simulink model "gm_max_frequency_index"  (R2020a)
settings: Solver=FixedStepDiscrete  StartTime=0.0  StopTime=1e-2  RelTol=1e-3
model workspace (MAT data in the model file):
  amplitud = 2047
  fft_length = 32
  samples_per_period = 3
  sampling_time = 1e-06
libraries: simulink x384, dspsrcs4 x1, dsphdlxfrm x1, dspstat3 x1, hdlsllib x1
(part 2 of 18)

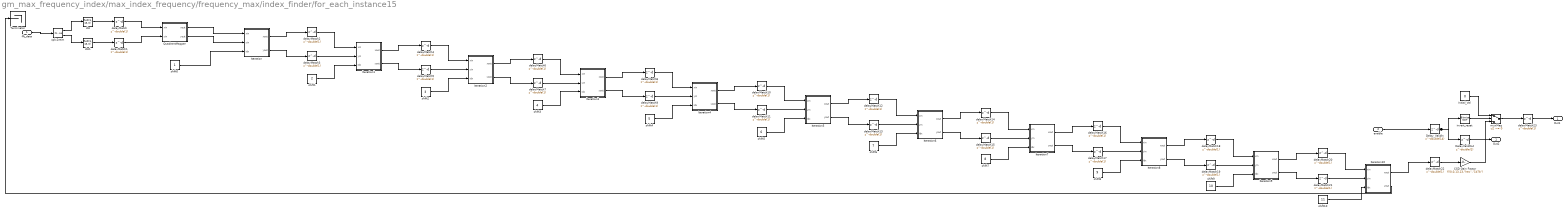
== system gm_max_frequency_index/max_index_frequency/frequency_max/index_finder/for_each_instance15 ==
  fft_data : Inport  OutDataTypeStr=fixdt(1, 12, 0)  PortDimensions=1  SampleTime=3.2e-05
      settings: SignalType=complex
  enable : Inport  Port=2  OutDataTypeStr=boolean  PortDimensions=1  SampleTime=3.2e-05
  CSD Gain Factor : Gain  Gain="fi(0,0,13,13,\"hex\",\"1b7b\")"  ParamDataTypeStr=fixdt(0, 13, 13)  OutDataTypeStr=fixdt(1, 13, 0)  SampleTime=3.2e-05
  DelayValidOut : Delay  DelayLength=double(1)  InitialCondition=0  SampleTime=3.2e-05
  Delay_ValidIn : Delay  DelayLength=double(14)  InitialCondition=0  SampleTime=3.2e-05
  Initial_Val : Constant  Value=0  OutDataTypeStr=fixdt(1, 13, 0)  SampleTime=3.2e-05
  Iteration : Subsystem
  Iteration1 : Subsystem
  Iteration10 : Subsystem
  Iteration2 : Subsystem
  Iteration3 : Subsystem
  Iteration4 : Subsystem
  Iteration5 : Subsystem
  Iteration6 : Subsystem
  Iteration7 : Subsystem
  Iteration8 : Subsystem
  Iteration9 : Subsystem
  QuadrantMapper : Subsystem
  Terminator : Terminator
  cplx2reim : ComplexToRealImag  SampleTime=3.2e-05
  delayMatch{,1..23} (24 alike) : Delay  DelayLength=double(1)  InitialCondition=0  SampleTime=3.2e-05
  dtc : DataTypeConversion  OutDataTypeStr=fixdt(1, 13, 0)  SampleTime=3.2e-05
  dtc1 : DataTypeConversion  OutDataTypeStr=fixdt(1, 13, 0)  SampleTime=3.2e-05
  invert_reset : simulink/Logic and Bit Operations/Bitwise Operator  logicop=NOT  UseBitMask=off  BitMask=double(0)  BitMaskRealWorld=Real World Value
  muxMag : Switch  Criteria=u2 ~= 0  Threshold=double(0)  OutDataTypeStr=fixdt(1, 13, 0)  SampleTime=3.2e-05
  shift0 : Constant  VectorParams1D=off  OutDataTypeStr=fixdt(0, 5, 0)  SampleTime=3.2e-05
  shift1 : Constant  Value=2  VectorParams1D=off  OutDataTypeStr=fixdt(0, 5, 0)  SampleTime=3.2e-05
  shift10 : Constant  Value=11  VectorParams1D=off  OutDataTypeStr=fixdt(0, 5, 0)  SampleTime=3.2e-05
  shift2 : Constant  Value=3  VectorParams1D=off  OutDataTypeStr=fixdt(0, 5, 0)  SampleTime=3.2e-05
  shift3 : Constant  Value=4  VectorParams1D=off  OutDataTypeStr=fixdt(0, 5, 0)  SampleTime=3.2e-05
  shift4 : Constant  Value=5  VectorParams1D=off  OutDataTypeStr=fixdt(0, 5, 0)  SampleTime=3.2e-05
  shift5 : Constant  Value=6  VectorParams1D=off  OutDataTypeStr=fixdt(0, 5, 0)  SampleTime=3.2e-05
  shift6 : Constant  Value=7  VectorParams1D=off  OutDataTypeStr=fixdt(0, 5, 0)  SampleTime=3.2e-05
  shift7 : Constant  Value=8  VectorParams1D=off  OutDataTypeStr=fixdt(0, 5, 0)  SampleTime=3.2e-05
  shift8 : Constant  Value=9  VectorParams1D=off  OutDataTypeStr=fixdt(0, 5, 0)  SampleTime=3.2e-05
  shift9 : Constant  Value=10  VectorParams1D=off  OutDataTypeStr=fixdt(0, 5, 0)  SampleTime=3.2e-05
  Out1 : Outport
  Out2 : Outport  Port=2  VectorParamsAs1DForOutWhenUnconnected=off
  wires:
  muxMag/1 -> delayMatch23/1
  invert_reset/1 -> muxMag/2
  CSD Gain Factor/1 -> muxMag/3
  Initial_Val/1 -> muxMag/1
  Iteration10/1(xout) -> delayMatch22/1
  shift10/1 -> Iteration10/3(idx)
  Iteration10/2(yout) -> Terminator/1
  Iteration9/2(yout) -> delayMatch21/1
  Iteration9/1(xout) -> delayMatch20/1
  shift9/1 -> Iteration9/3(idx)
  Iteration8/2(yout) -> delayMatch19/1
  Iteration8/1(xout) -> delayMatch18/1
  shift8/1 -> Iteration8/3(idx)
  Iteration7/2(yout) -> delayMatch17/1
  Iteration7/1(xout) -> delayMatch16/1
  shift7/1 -> Iteration7/3(idx)
  Iteration6/2(yout) -> delayMatch15/1
  Iteration6/1(xout) -> delayMatch14/1
  shift6/1 -> Iteration6/3(idx)
  Iteration5/2(yout) -> delayMatch13/1
  Iteration5/1(xout) -> delayMatch12/1
  shift5/1 -> Iteration5/3(idx)
  Iteration4/2(yout) -> delayMatch11/1
  Iteration4/1(xout) -> delayMatch10/1
  shift4/1 -> Iteration4/3(idx)
  Iteration3/2(yout) -> delayMatch9/1
  Iteration3/1(xout) -> delayMatch8/1
  shift3/1 -> Iteration3/3(idx)
  Iteration2/2(yout) -> delayMatch7/1
  Iteration2/1(xout) -> delayMatch6/1
  shift2/1 -> Iteration2/3(idx)
  Iteration1/2(yout) -> delayMatch5/1
  Iteration1/1(xout) -> delayMatch4/1
  shift1/1 -> Iteration1/3(idx)
  Iteration/2(yout) -> delayMatch3/1
  Iteration/1(xout) -> delayMatch2/1
  shift0/1 -> Iteration/3(idx)
  dtc1/1 -> delayMatch1/1
  dtc/1 -> delayMatch/1
  cplx2reim/2 -> dtc1/1
  cplx2reim/1 -> dtc/1
  enable/1 -> Delay_ValidIn/1
  fft_data/1 -> cplx2reim/1
  delayMatch23/1 -> Out1/1
  Delay_ValidIn/1 -> invert_reset/1, DelayValidOut/1
  QuadrantMapper/2(yout) -> Iteration/2(yin)
  QuadrantMapper/1(xout) -> Iteration/1(xin)
  delayMatch1/1 -> QuadrantMapper/2(yin)
  delayMatch/1 -> QuadrantMapper/1(xin)
  delayMatch22/1 -> CSD Gain Factor/1
  delayMatch21/1 -> Iteration10/2(yin)
  delayMatch20/1 -> Iteration10/1(xin)
  delayMatch19/1 -> Iteration9/2(yin)
  delayMatch18/1 -> Iteration9/1(xin)
  delayMatch17/1 -> Iteration8/2(yin)
  delayMatch16/1 -> Iteration8/1(xin)
  delayMatch15/1 -> Iteration7/2(yin)
  delayMatch14/1 -> Iteration7/1(xin)
  delayMatch13/1 -> Iteration6/2(yin)
  delayMatch12/1 -> Iteration6/1(xin)
  delayMatch11/1 -> Iteration5/2(yin)
  delayMatch10/1 -> Iteration5/1(xin)
  delayMatch9/1 -> Iteration4/2(yin)
  delayMatch8/1 -> Iteration4/1(xin)
  delayMatch7/1 -> Iteration3/2(yin)
  delayMatch6/1 -> Iteration3/1(xin)
  delayMatch5/1 -> Iteration2/2(yin)
  delayMatch4/1 -> Iteration2/1(xin)
  delayMatch3/1 -> Iteration1/2(yin)
  delayMatch2/1 -> Iteration1/1(xin)
  DelayValidOut/1 -> Out2/1

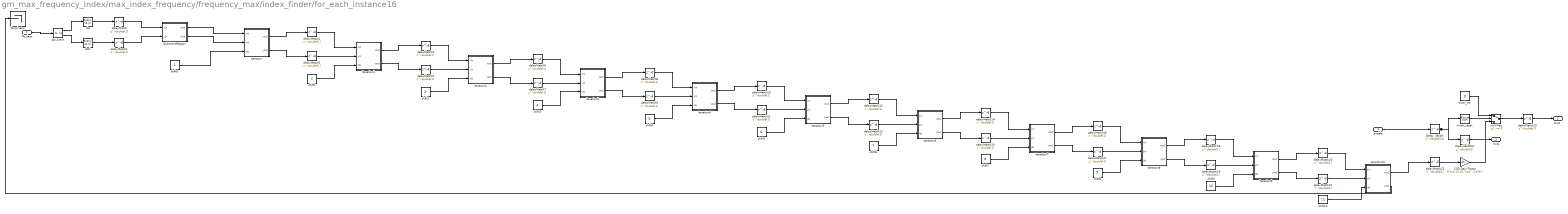
== system gm_max_frequency_index/max_index_frequency/frequency_max/index_finder/for_each_instance16 ==
  fft_data : Inport  OutDataTypeStr=fixdt(1, 12, 0)  PortDimensions=1  SampleTime=3.2e-05
      settings: SignalType=complex
  enable : Inport  Port=2  OutDataTypeStr=boolean  PortDimensions=1  SampleTime=3.2e-05
  CSD Gain Factor : Gain  Gain="fi(0,0,13,13,\"hex\",\"1b7b\")"  ParamDataTypeStr=fixdt(0, 13, 13)  OutDataTypeStr=fixdt(1, 13, 0)  SampleTime=3.2e-05
  DelayValidOut : Delay  DelayLength=double(1)  InitialCondition=0  SampleTime=3.2e-05
  Delay_ValidIn : Delay  DelayLength=double(14)  InitialCondition=0  SampleTime=3.2e-05
  Initial_Val : Constant  Value=0  OutDataTypeStr=fixdt(1, 13, 0)  SampleTime=3.2e-05
  Iteration : Subsystem
  Iteration1 : Subsystem
  Iteration10 : Subsystem
  Iteration2 : Subsystem
  Iteration3 : Subsystem
  Iteration4 : Subsystem
  Iteration5 : Subsystem
  Iteration6 : Subsystem
  Iteration7 : Subsystem
  Iteration8 : Subsystem
  Iteration9 : Subsystem
  QuadrantMapper : Subsystem
  Terminator : Terminator
  cplx2reim : ComplexToRealImag  SampleTime=3.2e-05
  delayMatch{,1..23} (24 alike) : Delay  DelayLength=double(1)  InitialCondition=0  SampleTime=3.2e-05
  dtc : DataTypeConversion  OutDataTypeStr=fixdt(1, 13, 0)  SampleTime=3.2e-05
  dtc1 : DataTypeConversion  OutDataTypeStr=fixdt(1, 13, 0)  SampleTime=3.2e-05
  invert_reset : simulink/Logic and Bit Operations/Bitwise Operator  logicop=NOT  UseBitMask=off  BitMask=double(0)  BitMaskRealWorld=Real World Value
  muxMag : Switch  Criteria=u2 ~= 0  Threshold=double(0)  OutDataTypeStr=fixdt(1, 13, 0)  SampleTime=3.2e-05
  shift0 : Constant  VectorParams1D=off  OutDataTypeStr=fixdt(0, 5, 0)  SampleTime=3.2e-05
  shift1 : Constant  Value=2  VectorParams1D=off  OutDataTypeStr=fixdt(0, 5, 0)  SampleTime=3.2e-05
  shift10 : Constant  Value=11  VectorParams1D=off  OutDataTypeStr=fixdt(0, 5, 0)  SampleTime=3.2e-05
  shift2 : Constant  Value=3  VectorParams1D=off  OutDataTypeStr=fixdt(0, 5, 0)  SampleTime=3.2e-05
  shift3 : Constant  Value=4  VectorParams1D=off  OutDataTypeStr=fixdt(0, 5, 0)  SampleTime=3.2e-05
  shift4 : Constant  Value=5  VectorParams1D=off  OutDataTypeStr=fixdt(0, 5, 0)  SampleTime=3.2e-05
  shift5 : Constant  Value=6  VectorParams1D=off  OutDataTypeStr=fixdt(0, 5, 0)  SampleTime=3.2e-05
  shift6 : Constant  Value=7  VectorParams1D=off  OutDataTypeStr=fixdt(0, 5, 0)  SampleTime=3.2e-05
  shift7 : Constant  Value=8  VectorParams1D=off  OutDataTypeStr=fixdt(0, 5, 0)  SampleTime=3.2e-05
  shift8 : Constant  Value=9  VectorParams1D=off  OutDataTypeStr=fixdt(0, 5, 0)  SampleTime=3.2e-05
  shift9 : Constant  Value=10  VectorParams1D=off  OutDataTypeStr=fixdt(0, 5, 0)  SampleTime=3.2e-05
  Out1 : Outport
  Out2 : Outport  Port=2  VectorParamsAs1DForOutWhenUnconnected=off
  wires:
  muxMag/1 -> delayMatch23/1
  invert_reset/1 -> muxMag/2
  CSD Gain Factor/1 -> muxMag/3
  Initial_Val/1 -> muxMag/1
  Iteration10/1(xout) -> delayMatch22/1
  shift10/1 -> Iteration10/3(idx)
  Iteration10/2(yout) -> Terminator/1
  Iteration9/2(yout) -> delayMatch21/1
  Iteration9/1(xout) -> delayMatch20/1
  shift9/1 -> Iteration9/3(idx)
  Iteration8/2(yout) -> delayMatch19/1
  Iteration8/1(xout) -> delayMatch18/1
  shift8/1 -> Iteration8/3(idx)
  Iteration7/2(yout) -> delayMatch17/1
  Iteration7/1(xout) -> delayMatch16/1
  shift7/1 -> Iteration7/3(idx)
  Iteration6/2(yout) -> delayMatch15/1
  Iteration6/1(xout) -> delayMatch14/1
  shift6/1 -> Iteration6/3(idx)
  Iteration5/2(yout) -> delayMatch13/1
  Iteration5/1(xout) -> delayMatch12/1
  shift5/1 -> Iteration5/3(idx)
  Iteration4/2(yout) -> delayMatch11/1
  Iteration4/1(xout) -> delayMatch10/1
  shift4/1 -> Iteration4/3(idx)
  Iteration3/2(yout) -> delayMatch9/1
  Iteration3/1(xout) -> delayMatch8/1
  shift3/1 -> Iteration3/3(idx)
  Iteration2/2(yout) -> delayMatch7/1
  Iteration2/1(xout) -> delayMatch6/1
  shift2/1 -> Iteration2/3(idx)
  Iteration1/2(yout) -> delayMatch5/1
  Iteration1/1(xout) -> delayMatch4/1
  shift1/1 -> Iteration1/3(idx)
  Iteration/2(yout) -> delayMatch3/1
  Iteration/1(xout) -> delayMatch2/1
  shift0/1 -> Iteration/3(idx)
  dtc1/1 -> delayMatch1/1
  dtc/1 -> delayMatch/1
  cplx2reim/2 -> dtc1/1
  cplx2reim/1 -> dtc/1
  enable/1 -> Delay_ValidIn/1
  fft_data/1 -> cplx2reim/1
  delayMatch23/1 -> Out1/1
  Delay_ValidIn/1 -> invert_reset/1, DelayValidOut/1
  QuadrantMapper/2(yout) -> Iteration/2(yin)
  QuadrantMapper/1(xout) -> Iteration/1(xin)
  delayMatch1/1 -> QuadrantMapper/2(yin)
  delayMatch/1 -> QuadrantMapper/1(xin)
  delayMatch22/1 -> CSD Gain Factor/1
  delayMatch21/1 -> Iteration10/2(yin)
  delayMatch20/1 -> Iteration10/1(xin)
  delayMatch19/1 -> Iteration9/2(yin)
  delayMatch18/1 -> Iteration9/1(xin)
  delayMatch17/1 -> Iteration8/2(yin)
  delayMatch16/1 -> Iteration8/1(xin)
  delayMatch15/1 -> Iteration7/2(yin)
  delayMatch14/1 -> Iteration7/1(xin)
  delayMatch13/1 -> Iteration6/2(yin)
  delayMatch12/1 -> Iteration6/1(xin)
  delayMatch11/1 -> Iteration5/2(yin)
  delayMatch10/1 -> Iteration5/1(xin)
  delayMatch9/1 -> Iteration4/2(yin)
  delayMatch8/1 -> Iteration4/1(xin)
  delayMatch7/1 -> Iteration3/2(yin)
  delayMatch6/1 -> Iteration3/1(xin)
  delayMatch5/1 -> Iteration2/2(yin)
  delayMatch4/1 -> Iteration2/1(xin)
  delayMatch3/1 -> Iteration1/2(yin)
  delayMatch2/1 -> Iteration1/1(xin)
  DelayValidOut/1 -> Out2/1

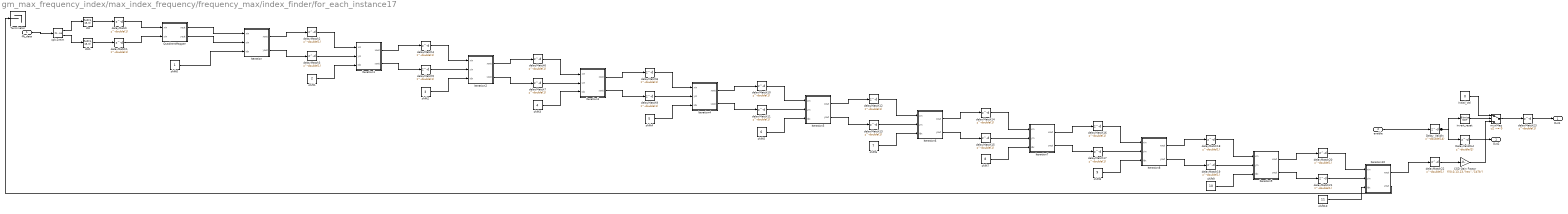
== system gm_max_frequency_index/max_index_frequency/frequency_max/index_finder/for_each_instance17 ==
  fft_data : Inport  OutDataTypeStr=fixdt(1, 12, 0)  PortDimensions=1  SampleTime=3.2e-05
      settings: SignalType=complex
  enable : Inport  Port=2  OutDataTypeStr=boolean  PortDimensions=1  SampleTime=3.2e-05
  CSD Gain Factor : Gain  Gain="fi(0,0,13,13,\"hex\",\"1b7b\")"  ParamDataTypeStr=fixdt(0, 13, 13)  OutDataTypeStr=fixdt(1, 13, 0)  SampleTime=3.2e-05
  DelayValidOut : Delay  DelayLength=double(1)  InitialCondition=0  SampleTime=3.2e-05
  Delay_ValidIn : Delay  DelayLength=double(14)  InitialCondition=0  SampleTime=3.2e-05
  Initial_Val : Constant  Value=0  OutDataTypeStr=fixdt(1, 13, 0)  SampleTime=3.2e-05
  Iteration : Subsystem
  Iteration1 : Subsystem
  Iteration10 : Subsystem
  Iteration2 : Subsystem
  Iteration3 : Subsystem
  Iteration4 : Subsystem
  Iteration5 : Subsystem
  Iteration6 : Subsystem
  Iteration7 : Subsystem
  Iteration8 : Subsystem
  Iteration9 : Subsystem
  QuadrantMapper : Subsystem
  Terminator : Terminator
  cplx2reim : ComplexToRealImag  SampleTime=3.2e-05
  delayMatch{,1..23} (24 alike) : Delay  DelayLength=double(1)  InitialCondition=0  SampleTime=3.2e-05
  dtc : DataTypeConversion  OutDataTypeStr=fixdt(1, 13, 0)  SampleTime=3.2e-05
  dtc1 : DataTypeConversion  OutDataTypeStr=fixdt(1, 13, 0)  SampleTime=3.2e-05
  invert_reset : simulink/Logic and Bit Operations/Bitwise Operator  logicop=NOT  UseBitMask=off  BitMask=double(0)  BitMaskRealWorld=Real World Value
  muxMag : Switch  Criteria=u2 ~= 0  Threshold=double(0)  OutDataTypeStr=fixdt(1, 13, 0)  SampleTime=3.2e-05
  shift0 : Constant  VectorParams1D=off  OutDataTypeStr=fixdt(0, 5, 0)  SampleTime=3.2e-05
  shift1 : Constant  Value=2  VectorParams1D=off  OutDataTypeStr=fixdt(0, 5, 0)  SampleTime=3.2e-05
  shift10 : Constant  Value=11  VectorParams1D=off  OutDataTypeStr=fixdt(0, 5, 0)  SampleTime=3.2e-05
  shift2 : Constant  Value=3  VectorParams1D=off  OutDataTypeStr=fixdt(0, 5, 0)  SampleTime=3.2e-05
  shift3 : Constant  Value=4  VectorParams1D=off  OutDataTypeStr=fixdt(0, 5, 0)  SampleTime=3.2e-05
  shift4 : Constant  Value=5  VectorParams1D=off  OutDataTypeStr=fixdt(0, 5, 0)  SampleTime=3.2e-05
  shift5 : Constant  Value=6  VectorParams1D=off  OutDataTypeStr=fixdt(0, 5, 0)  SampleTime=3.2e-05
  shift6 : Constant  Value=7  VectorParams1D=off  OutDataTypeStr=fixdt(0, 5, 0)  SampleTime=3.2e-05
  shift7 : Constant  Value=8  VectorParams1D=off  OutDataTypeStr=fixdt(0, 5, 0)  SampleTime=3.2e-05
  shift8 : Constant  Value=9  VectorParams1D=off  OutDataTypeStr=fixdt(0, 5, 0)  SampleTime=3.2e-05
  shift9 : Constant  Value=10  VectorParams1D=off  OutDataTypeStr=fixdt(0, 5, 0)  SampleTime=3.2e-05
  Out1 : Outport
  Out2 : Outport  Port=2  VectorParamsAs1DForOutWhenUnconnected=off
  wires:
  muxMag/1 -> delayMatch23/1
  invert_reset/1 -> muxMag/2
  CSD Gain Factor/1 -> muxMag/3
  Initial_Val/1 -> muxMag/1
  Iteration10/1(xout) -> delayMatch22/1
  shift10/1 -> Iteration10/3(idx)
  Iteration10/2(yout) -> Terminator/1
  Iteration9/2(yout) -> delayMatch21/1
  Iteration9/1(xout) -> delayMatch20/1
  shift9/1 -> Iteration9/3(idx)
  Iteration8/2(yout) -> delayMatch19/1
  Iteration8/1(xout) -> delayMatch18/1
  shift8/1 -> Iteration8/3(idx)
  Iteration7/2(yout) -> delayMatch17/1
  Iteration7/1(xout) -> delayMatch16/1
  shift7/1 -> Iteration7/3(idx)
  Iteration6/2(yout) -> delayMatch15/1
  Iteration6/1(xout) -> delayMatch14/1
  shift6/1 -> Iteration6/3(idx)
  Iteration5/2(yout) -> delayMatch13/1
  Iteration5/1(xout) -> delayMatch12/1
  shift5/1 -> Iteration5/3(idx)
  Iteration4/2(yout) -> delayMatch11/1
  Iteration4/1(xout) -> delayMatch10/1
  shift4/1 -> Iteration4/3(idx)
  Iteration3/2(yout) -> delayMatch9/1
  Iteration3/1(xout) -> delayMatch8/1
  shift3/1 -> Iteration3/3(idx)
  Iteration2/2(yout) -> delayMatch7/1
  Iteration2/1(xout) -> delayMatch6/1
  shift2/1 -> Iteration2/3(idx)
  Iteration1/2(yout) -> delayMatch5/1
  Iteration1/1(xout) -> delayMatch4/1
  shift1/1 -> Iteration1/3(idx)
  Iteration/2(yout) -> delayMatch3/1
  Iteration/1(xout) -> delayMatch2/1
  shift0/1 -> Iteration/3(idx)
  dtc1/1 -> delayMatch1/1
  dtc/1 -> delayMatch/1
  cplx2reim/2 -> dtc1/1
  cplx2reim/1 -> dtc/1
  enable/1 -> Delay_ValidIn/1
  fft_data/1 -> cplx2reim/1
  delayMatch23/1 -> Out1/1
  Delay_ValidIn/1 -> invert_reset/1, DelayValidOut/1
  QuadrantMapper/2(yout) -> Iteration/2(yin)
  QuadrantMapper/1(xout) -> Iteration/1(xin)
  delayMatch1/1 -> QuadrantMapper/2(yin)
  delayMatch/1 -> QuadrantMapper/1(xin)
  delayMatch22/1 -> CSD Gain Factor/1
  delayMatch21/1 -> Iteration10/2(yin)
  delayMatch20/1 -> Iteration10/1(xin)
  delayMatch19/1 -> Iteration9/2(yin)
  delayMatch18/1 -> Iteration9/1(xin)
  delayMatch17/1 -> Iteration8/2(yin)
  delayMatch16/1 -> Iteration8/1(xin)
  delayMatch15/1 -> Iteration7/2(yin)
  delayMatch14/1 -> Iteration7/1(xin)
  delayMatch13/1 -> Iteration6/2(yin)
  delayMatch12/1 -> Iteration6/1(xin)
  delayMatch11/1 -> Iteration5/2(yin)
  delayMatch10/1 -> Iteration5/1(xin)
  delayMatch9/1 -> Iteration4/2(yin)
  delayMatch8/1 -> Iteration4/1(xin)
  delayMatch7/1 -> Iteration3/2(yin)
  delayMatch6/1 -> Iteration3/1(xin)
  delayMatch5/1 -> Iteration2/2(yin)
  delayMatch4/1 -> Iteration2/1(xin)
  delayMatch3/1 -> Iteration1/2(yin)
  delayMatch2/1 -> Iteration1/1(xin)
  DelayValidOut/1 -> Out2/1

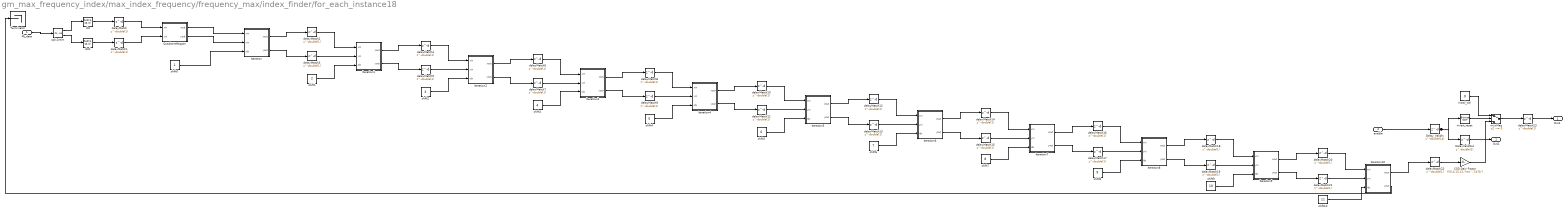
== system gm_max_frequency_index/max_index_frequency/frequency_max/index_finder/for_each_instance18 ==
  fft_data : Inport  OutDataTypeStr=fixdt(1, 12, 0)  PortDimensions=1  SampleTime=3.2e-05
      settings: SignalType=complex
  enable : Inport  Port=2  OutDataTypeStr=boolean  PortDimensions=1  SampleTime=3.2e-05
  CSD Gain Factor : Gain  Gain="fi(0,0,13,13,\"hex\",\"1b7b\")"  ParamDataTypeStr=fixdt(0, 13, 13)  OutDataTypeStr=fixdt(1, 13, 0)  SampleTime=3.2e-05
  DelayValidOut : Delay  DelayLength=double(1)  InitialCondition=0  SampleTime=3.2e-05
  Delay_ValidIn : Delay  DelayLength=double(14)  InitialCondition=0  SampleTime=3.2e-05
  Initial_Val : Constant  Value=0  OutDataTypeStr=fixdt(1, 13, 0)  SampleTime=3.2e-05
  Iteration : Subsystem
  Iteration1 : Subsystem
  Iteration10 : Subsystem
  Iteration2 : Subsystem
  Iteration3 : Subsystem
  Iteration4 : Subsystem
  Iteration5 : Subsystem
  Iteration6 : Subsystem
  Iteration7 : Subsystem
  Iteration8 : Subsystem
  Iteration9 : Subsystem
  QuadrantMapper : Subsystem
  Terminator : Terminator
  cplx2reim : ComplexToRealImag  SampleTime=3.2e-05
  delayMatch{,1..23} (24 alike) : Delay  DelayLength=double(1)  InitialCondition=0  SampleTime=3.2e-05
  dtc : DataTypeConversion  OutDataTypeStr=fixdt(1, 13, 0)  SampleTime=3.2e-05
  dtc1 : DataTypeConversion  OutDataTypeStr=fixdt(1, 13, 0)  SampleTime=3.2e-05
  invert_reset : simulink/Logic and Bit Operations/Bitwise Operator  logicop=NOT  UseBitMask=off  BitMask=double(0)  BitMaskRealWorld=Real World Value
  muxMag : Switch  Criteria=u2 ~= 0  Threshold=double(0)  OutDataTypeStr=fixdt(1, 13, 0)  SampleTime=3.2e-05
  shift0 : Constant  VectorParams1D=off  OutDataTypeStr=fixdt(0, 5, 0)  SampleTime=3.2e-05
  shift1 : Constant  Value=2  VectorParams1D=off  OutDataTypeStr=fixdt(0, 5, 0)  SampleTime=3.2e-05
  shift10 : Constant  Value=11  VectorParams1D=off  OutDataTypeStr=fixdt(0, 5, 0)  SampleTime=3.2e-05
  shift2 : Constant  Value=3  VectorParams1D=off  OutDataTypeStr=fixdt(0, 5, 0)  SampleTime=3.2e-05
  shift3 : Constant  Value=4  VectorParams1D=off  OutDataTypeStr=fixdt(0, 5, 0)  SampleTime=3.2e-05
  shift4 : Constant  Value=5  VectorParams1D=off  OutDataTypeStr=fixdt(0, 5, 0)  SampleTime=3.2e-05
  shift5 : Constant  Value=6  VectorParams1D=off  OutDataTypeStr=fixdt(0, 5, 0)  SampleTime=3.2e-05
  shift6 : Constant  Value=7  VectorParams1D=off  OutDataTypeStr=fixdt(0, 5, 0)  SampleTime=3.2e-05
  shift7 : Constant  Value=8  VectorParams1D=off  OutDataTypeStr=fixdt(0, 5, 0)  SampleTime=3.2e-05
  shift8 : Constant  Value=9  VectorParams1D=off  OutDataTypeStr=fixdt(0, 5, 0)  SampleTime=3.2e-05
  shift9 : Constant  Value=10  VectorParams1D=off  OutDataTypeStr=fixdt(0, 5, 0)  SampleTime=3.2e-05
  Out1 : Outport
  Out2 : Outport  Port=2  VectorParamsAs1DForOutWhenUnconnected=off
  wires:
  muxMag/1 -> delayMatch23/1
  invert_reset/1 -> muxMag/2
  CSD Gain Factor/1 -> muxMag/3
  Initial_Val/1 -> muxMag/1
  Iteration10/1(xout) -> delayMatch22/1
  shift10/1 -> Iteration10/3(idx)
  Iteration10/2(yout) -> Terminator/1
  Iteration9/2(yout) -> delayMatch21/1
  Iteration9/1(xout) -> delayMatch20/1
  shift9/1 -> Iteration9/3(idx)
  Iteration8/2(yout) -> delayMatch19/1
  Iteration8/1(xout) -> delayMatch18/1
  shift8/1 -> Iteration8/3(idx)
  Iteration7/2(yout) -> delayMatch17/1
  Iteration7/1(xout) -> delayMatch16/1
  shift7/1 -> Iteration7/3(idx)
  Iteration6/2(yout) -> delayMatch15/1
  Iteration6/1(xout) -> delayMatch14/1
  shift6/1 -> Iteration6/3(idx)
  Iteration5/2(yout) -> delayMatch13/1
  Iteration5/1(xout) -> delayMatch12/1
  shift5/1 -> Iteration5/3(idx)
  Iteration4/2(yout) -> delayMatch11/1
  Iteration4/1(xout) -> delayMatch10/1
  shift4/1 -> Iteration4/3(idx)
  Iteration3/2(yout) -> delayMatch9/1
  Iteration3/1(xout) -> delayMatch8/1
  shift3/1 -> Iteration3/3(idx)
  Iteration2/2(yout) -> delayMatch7/1
  Iteration2/1(xout) -> delayMatch6/1
  shift2/1 -> Iteration2/3(idx)
  Iteration1/2(yout) -> delayMatch5/1
  Iteration1/1(xout) -> delayMatch4/1
  shift1/1 -> Iteration1/3(idx)
  Iteration/2(yout) -> delayMatch3/1
  Iteration/1(xout) -> delayMatch2/1
  shift0/1 -> Iteration/3(idx)
  dtc1/1 -> delayMatch1/1
  dtc/1 -> delayMatch/1
  cplx2reim/2 -> dtc1/1
  cplx2reim/1 -> dtc/1
  enable/1 -> Delay_ValidIn/1
  fft_data/1 -> cplx2reim/1
  delayMatch23/1 -> Out1/1
  Delay_ValidIn/1 -> invert_reset/1, DelayValidOut/1
  QuadrantMapper/2(yout) -> Iteration/2(yin)
  QuadrantMapper/1(xout) -> Iteration/1(xin)
  delayMatch1/1 -> QuadrantMapper/2(yin)
  delayMatch/1 -> QuadrantMapper/1(xin)
  delayMatch22/1 -> CSD Gain Factor/1
  delayMatch21/1 -> Iteration10/2(yin)
  delayMatch20/1 -> Iteration10/1(xin)
  delayMatch19/1 -> Iteration9/2(yin)
  delayMatch18/1 -> Iteration9/1(xin)
  delayMatch17/1 -> Iteration8/2(yin)
  delayMatch16/1 -> Iteration8/1(xin)
  delayMatch15/1 -> Iteration7/2(yin)
  delayMatch14/1 -> Iteration7/1(xin)
  delayMatch13/1 -> Iteration6/2(yin)
  delayMatch12/1 -> Iteration6/1(xin)
  delayMatch11/1 -> Iteration5/2(yin)
  delayMatch10/1 -> Iteration5/1(xin)
  delayMatch9/1 -> Iteration4/2(yin)
  delayMatch8/1 -> Iteration4/1(xin)
  delayMatch7/1 -> Iteration3/2(yin)
  delayMatch6/1 -> Iteration3/1(xin)
  delayMatch5/1 -> Iteration2/2(yin)
  delayMatch4/1 -> Iteration2/1(xin)
  delayMatch3/1 -> Iteration1/2(yin)
  delayMatch2/1 -> Iteration1/1(xin)
  DelayValidOut/1 -> Out2/1

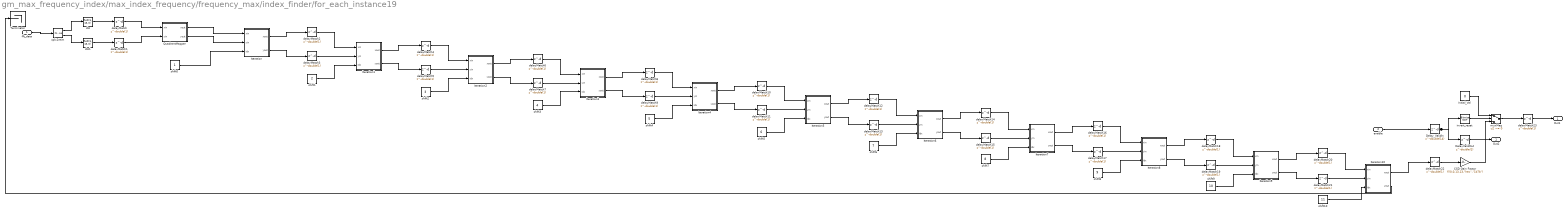
== system gm_max_frequency_index/max_index_frequency/frequency_max/index_finder/for_each_instance19 ==
  fft_data : Inport  OutDataTypeStr=fixdt(1, 12, 0)  PortDimensions=1  SampleTime=3.2e-05
      settings: SignalType=complex
  enable : Inport  Port=2  OutDataTypeStr=boolean  PortDimensions=1  SampleTime=3.2e-05
  CSD Gain Factor : Gain  Gain="fi(0,0,13,13,\"hex\",\"1b7b\")"  ParamDataTypeStr=fixdt(0, 13, 13)  OutDataTypeStr=fixdt(1, 13, 0)  SampleTime=3.2e-05
  DelayValidOut : Delay  DelayLength=double(1)  InitialCondition=0  SampleTime=3.2e-05
  Delay_ValidIn : Delay  DelayLength=double(14)  InitialCondition=0  SampleTime=3.2e-05
  Initial_Val : Constant  Value=0  OutDataTypeStr=fixdt(1, 13, 0)  SampleTime=3.2e-05
  Iteration : Subsystem
  Iteration1 : Subsystem
  Iteration10 : Subsystem
  Iteration2 : Subsystem
  Iteration3 : Subsystem
  Iteration4 : Subsystem
  Iteration5 : Subsystem
  Iteration6 : Subsystem
  Iteration7 : Subsystem
  Iteration8 : Subsystem
  Iteration9 : Subsystem
  QuadrantMapper : Subsystem
  Terminator : Terminator
  cplx2reim : ComplexToRealImag  SampleTime=3.2e-05
  delayMatch{,1..23} (24 alike) : Delay  DelayLength=double(1)  InitialCondition=0  SampleTime=3.2e-05
  dtc : DataTypeConversion  OutDataTypeStr=fixdt(1, 13, 0)  SampleTime=3.2e-05
  dtc1 : DataTypeConversion  OutDataTypeStr=fixdt(1, 13, 0)  SampleTime=3.2e-05
  invert_reset : simulink/Logic and Bit Operations/Bitwise Operator  logicop=NOT  UseBitMask=off  BitMask=double(0)  BitMaskRealWorld=Real World Value
  muxMag : Switch  Criteria=u2 ~= 0  Threshold=double(0)  OutDataTypeStr=fixdt(1, 13, 0)  SampleTime=3.2e-05
  shift0 : Constant  VectorParams1D=off  OutDataTypeStr=fixdt(0, 5, 0)  SampleTime=3.2e-05
  shift1 : Constant  Value=2  VectorParams1D=off  OutDataTypeStr=fixdt(0, 5, 0)  SampleTime=3.2e-05
  shift10 : Constant  Value=11  VectorParams1D=off  OutDataTypeStr=fixdt(0, 5, 0)  SampleTime=3.2e-05
  shift2 : Constant  Value=3  VectorParams1D=off  OutDataTypeStr=fixdt(0, 5, 0)  SampleTime=3.2e-05
  shift3 : Constant  Value=4  VectorParams1D=off  OutDataTypeStr=fixdt(0, 5, 0)  SampleTime=3.2e-05
  shift4 : Constant  Value=5  VectorParams1D=off  OutDataTypeStr=fixdt(0, 5, 0)  SampleTime=3.2e-05
  shift5 : Constant  Value=6  VectorParams1D=off  OutDataTypeStr=fixdt(0, 5, 0)  SampleTime=3.2e-05
  shift6 : Constant  Value=7  VectorParams1D=off  OutDataTypeStr=fixdt(0, 5, 0)  SampleTime=3.2e-05
  shift7 : Constant  Value=8  VectorParams1D=off  OutDataTypeStr=fixdt(0, 5, 0)  SampleTime=3.2e-05
  shift8 : Constant  Value=9  VectorParams1D=off  OutDataTypeStr=fixdt(0, 5, 0)  SampleTime=3.2e-05
  shift9 : Constant  Value=10  VectorParams1D=off  OutDataTypeStr=fixdt(0, 5, 0)  SampleTime=3.2e-05
  Out1 : Outport
  Out2 : Outport  Port=2  VectorParamsAs1DForOutWhenUnconnected=off
  wires:
  muxMag/1 -> delayMatch23/1
  invert_reset/1 -> muxMag/2
  CSD Gain Factor/1 -> muxMag/3
  Initial_Val/1 -> muxMag/1
  Iteration10/1(xout) -> delayMatch22/1
  shift10/1 -> Iteration10/3(idx)
  Iteration10/2(yout) -> Terminator/1
  Iteration9/2(yout) -> delayMatch21/1
  Iteration9/1(xout) -> delayMatch20/1
  shift9/1 -> Iteration9/3(idx)
  Iteration8/2(yout) -> delayMatch19/1
  Iteration8/1(xout) -> delayMatch18/1
  shift8/1 -> Iteration8/3(idx)
  Iteration7/2(yout) -> delayMatch17/1
  Iteration7/1(xout) -> delayMatch16/1
  shift7/1 -> Iteration7/3(idx)
  Iteration6/2(yout) -> delayMatch15/1
  Iteration6/1(xout) -> delayMatch14/1
  shift6/1 -> Iteration6/3(idx)
  Iteration5/2(yout) -> delayMatch13/1
  Iteration5/1(xout) -> delayMatch12/1
  shift5/1 -> Iteration5/3(idx)
  Iteration4/2(yout) -> delayMatch11/1
  Iteration4/1(xout) -> delayMatch10/1
  shift4/1 -> Iteration4/3(idx)
  Iteration3/2(yout) -> delayMatch9/1
  Iteration3/1(xout) -> delayMatch8/1
  shift3/1 -> Iteration3/3(idx)
  Iteration2/2(yout) -> delayMatch7/1
  Iteration2/1(xout) -> delayMatch6/1
  shift2/1 -> Iteration2/3(idx)
  Iteration1/2(yout) -> delayMatch5/1
  Iteration1/1(xout) -> delayMatch4/1
  shift1/1 -> Iteration1/3(idx)
  Iteration/2(yout) -> delayMatch3/1
  Iteration/1(xout) -> delayMatch2/1
  shift0/1 -> Iteration/3(idx)
  dtc1/1 -> delayMatch1/1
  dtc/1 -> delayMatch/1
  cplx2reim/2 -> dtc1/1
  cplx2reim/1 -> dtc/1
  enable/1 -> Delay_ValidIn/1
  fft_data/1 -> cplx2reim/1
  delayMatch23/1 -> Out1/1
  Delay_ValidIn/1 -> invert_reset/1, DelayValidOut/1
  QuadrantMapper/2(yout) -> Iteration/2(yin)
  QuadrantMapper/1(xout) -> Iteration/1(xin)
  delayMatch1/1 -> QuadrantMapper/2(yin)
  delayMatch/1 -> QuadrantMapper/1(xin)
  delayMatch22/1 -> CSD Gain Factor/1
  delayMatch21/1 -> Iteration10/2(yin)
  delayMatch20/1 -> Iteration10/1(xin)
  delayMatch19/1 -> Iteration9/2(yin)
  delayMatch18/1 -> Iteration9/1(xin)
  delayMatch17/1 -> Iteration8/2(yin)
  delayMatch16/1 -> Iteration8/1(xin)
  delayMatch15/1 -> Iteration7/2(yin)
  delayMatch14/1 -> Iteration7/1(xin)
  delayMatch13/1 -> Iteration6/2(yin)
  delayMatch12/1 -> Iteration6/1(xin)
  delayMatch11/1 -> Iteration5/2(yin)
  delayMatch10/1 -> Iteration5/1(xin)
  delayMatch9/1 -> Iteration4/2(yin)
  delayMatch8/1 -> Iteration4/1(xin)
  delayMatch7/1 -> Iteration3/2(yin)
  delayMatch6/1 -> Iteration3/1(xin)
  delayMatch5/1 -> Iteration2/2(yin)
  delayMatch4/1 -> Iteration2/1(xin)
  delayMatch3/1 -> Iteration1/2(yin)
  delayMatch2/1 -> Iteration1/1(xin)
  DelayValidOut/1 -> Out2/1

== system gm_max_frequency_index/max_index_frequency/frequency_max/index_finder/for_each_instance2 ==
  fft_data : Inport  OutDataTypeStr=fixdt(1, 12, 0)  PortDimensions=1  SampleTime=3.2e-05
      settings: SignalType=complex
  enable : Inport  Port=2  OutDataTypeStr=boolean  PortDimensions=1  SampleTime=3.2e-05
  CSD Gain Factor : Gain  Gain="fi(0,0,13,13,\"hex\",\"1b7b\")"  ParamDataTypeStr=fixdt(0, 13, 13)  OutDataTypeStr=fixdt(1, 13, 0)  SampleTime=3.2e-05
  DelayValidOut : Delay  DelayLength=double(1)  InitialCondition=0  SampleTime=3.2e-05
  Delay_ValidIn : Delay  DelayLength=double(14)  InitialCondition=0  SampleTime=3.2e-05
  Initial_Val : Constant  Value=0  OutDataTypeStr=fixdt(1, 13, 0)  SampleTime=3.2e-05
  Iteration : Subsystem
  Iteration1 : Subsystem
  Iteration10 : Subsystem
  Iteration2 : Subsystem
  Iteration3 : Subsystem
  Iteration4 : Subsystem
  Iteration5 : Subsystem
  Iteration6 : Subsystem
  Iteration7 : Subsystem
  Iteration8 : Subsystem
  Iteration9 : Subsystem
  QuadrantMapper : Subsystem
  Terminator : Terminator
  cplx2reim : ComplexToRealImag  SampleTime=3.2e-05
  delayMatch{,1..23} (24 alike) : Delay  DelayLength=double(1)  InitialCondition=0  SampleTime=3.2e-05
  dtc : DataTypeConversion  OutDataTypeStr=fixdt(1, 13, 0)  SampleTime=3.2e-05
  dtc1 : DataTypeConversion  OutDataTypeStr=fixdt(1, 13, 0)  SampleTime=3.2e-05
  invert_reset : simulink/Logic and Bit Operations/Bitwise Operator  logicop=NOT  UseBitMask=off  BitMask=double(0)  BitMaskRealWorld=Real World Value
  muxMag : Switch  Criteria=u2 ~= 0  Threshold=double(0)  OutDataTypeStr=fixdt(1, 13, 0)  SampleTime=3.2e-05
  shift0 : Constant  VectorParams1D=off  OutDataTypeStr=fixdt(0, 5, 0)  SampleTime=3.2e-05
  shift1 : Constant  Value=2  VectorParams1D=off  OutDataTypeStr=fixdt(0, 5, 0)  SampleTime=3.2e-05
  shift10 : Constant  Value=11  VectorParams1D=off  OutDataTypeStr=fixdt(0, 5, 0)  SampleTime=3.2e-05
  shift2 : Constant  Value=3  VectorParams1D=off  OutDataTypeStr=fixdt(0, 5, 0)  SampleTime=3.2e-05
  shift3 : Constant  Value=4  VectorParams1D=off  OutDataTypeStr=fixdt(0, 5, 0)  SampleTime=3.2e-05
  shift4 : Constant  Value=5  VectorParams1D=off  OutDataTypeStr=fixdt(0, 5, 0)  SampleTime=3.2e-05
  shift5 : Constant  Value=6  VectorParams1D=off  OutDataTypeStr=fixdt(0, 5, 0)  SampleTime=3.2e-05
  shift6 : Constant  Value=7  VectorParams1D=off  OutDataTypeStr=fixdt(0, 5, 0)  SampleTime=3.2e-05
  shift7 : Constant  Value=8  VectorParams1D=off  OutDataTypeStr=fixdt(0, 5, 0)  SampleTime=3.2e-05
  shift8 : Constant  Value=9  VectorParams1D=off  OutDataTypeStr=fixdt(0, 5, 0)  SampleTime=3.2e-05
  shift9 : Constant  Value=10  VectorParams1D=off  OutDataTypeStr=fixdt(0, 5, 0)  SampleTime=3.2e-05
  Out1 : Outport
  Out2 : Outport  Port=2  VectorParamsAs1DForOutWhenUnconnected=off
  wires:
  muxMag/1 -> delayMatch23/1
  invert_reset/1 -> muxMag/2
  CSD Gain Factor/1 -> muxMag/3
  Initial_Val/1 -> muxMag/1
  Iteration10/1(xout) -> delayMatch22/1
  shift10/1 -> Iteration10/3(idx)
  Iteration10/2(yout) -> Terminator/1
  Iteration9/2(yout) -> delayMatch21/1
  Iteration9/1(xout) -> delayMatch20/1
  shift9/1 -> Iteration9/3(idx)
  Iteration8/2(yout) -> delayMatch19/1
  Iteration8/1(xout) -> delayMatch18/1
  shift8/1 -> Iteration8/3(idx)
  Iteration7/2(yout) -> delayMatch17/1
  Iteration7/1(xout) -> delayMatch16/1
  shift7/1 -> Iteration7/3(idx)
  Iteration6/2(yout) -> delayMatch15/1
  Iteration6/1(xout) -> delayMatch14/1
  shift6/1 -> Iteration6/3(idx)
  Iteration5/2(yout) -> delayMatch13/1
  Iteration5/1(xout) -> delayMatch12/1
  shift5/1 -> Iteration5/3(idx)
  Iteration4/2(yout) -> delayMatch11/1
  Iteration4/1(xout) -> delayMatch10/1
  shift4/1 -> Iteration4/3(idx)
  Iteration3/2(yout) -> delayMatch9/1
  Iteration3/1(xout) -> delayMatch8/1
  shift3/1 -> Iteration3/3(idx)
  Iteration2/2(yout) -> delayMatch7/1
  Iteration2/1(xout) -> delayMatch6/1
  shift2/1 -> Iteration2/3(idx)
  Iteration1/2(yout) -> delayMatch5/1
  Iteration1/1(xout) -> delayMatch4/1
  shift1/1 -> Iteration1/3(idx)
  Iteration/2(yout) -> delayMatch3/1
  Iteration/1(xout) -> delayMatch2/1
  shift0/1 -> Iteration/3(idx)
  dtc1/1 -> delayMatch1/1
  dtc/1 -> delayMatch/1
  cplx2reim/2 -> dtc1/1
  cplx2reim/1 -> dtc/1
  enable/1 -> Delay_ValidIn/1
  fft_data/1 -> cplx2reim/1
  delayMatch23/1 -> Out1/1
  Delay_ValidIn/1 -> invert_reset/1, DelayValidOut/1
  QuadrantMapper/2(yout) -> Iteration/2(yin)
  QuadrantMapper/1(xout) -> Iteration/1(xin)
  delayMatch1/1 -> QuadrantMapper/2(yin)
  delayMatch/1 -> QuadrantMapper/1(xin)
  delayMatch22/1 -> CSD Gain Factor/1
  delayMatch21/1 -> Iteration10/2(yin)
  delayMatch20/1 -> Iteration10/1(xin)
  delayMatch19/1 -> Iteration9/2(yin)
  delayMatch18/1 -> Iteration9/1(xin)
  delayMatch17/1 -> Iteration8/2(yin)
  delayMatch16/1 -> Iteration8/1(xin)
  delayMatch15/1 -> Iteration7/2(yin)
  delayMatch14/1 -> Iteration7/1(xin)
  delayMatch13/1 -> Iteration6/2(yin)
  delayMatch12/1 -> Iteration6/1(xin)
  delayMatch11/1 -> Iteration5/2(yin)
  delayMatch10/1 -> Iteration5/1(xin)
  delayMatch9/1 -> Iteration4/2(yin)
  delayMatch8/1 -> Iteration4/1(xin)
  delayMatch7/1 -> Iteration3/2(yin)
  delayMatch6/1 -> Iteration3/1(xin)
  delayMatch5/1 -> Iteration2/2(yin)
  delayMatch4/1 -> Iteration2/1(xin)
  delayMatch3/1 -> Iteration1/2(yin)
  delayMatch2/1 -> Iteration1/1(xin)
  DelayValidOut/1 -> Out2/1

== system gm_max_frequency_index/max_index_frequency/frequency_max/index_finder/for_each_instance20 ==
  fft_data : Inport  OutDataTypeStr=fixdt(1, 12, 0)  PortDimensions=1  SampleTime=3.2e-05
      settings: SignalType=complex
  enable : Inport  Port=2  OutDataTypeStr=boolean  PortDimensions=1  SampleTime=3.2e-05
  CSD Gain Factor : Gain  Gain="fi(0,0,13,13,\"hex\",\"1b7b\")"  ParamDataTypeStr=fixdt(0, 13, 13)  OutDataTypeStr=fixdt(1, 13, 0)  SampleTime=3.2e-05
  DelayValidOut : Delay  DelayLength=double(1)  InitialCondition=0  SampleTime=3.2e-05
  Delay_ValidIn : Delay  DelayLength=double(14)  InitialCondition=0  SampleTime=3.2e-05
  Initial_Val : Constant  Value=0  OutDataTypeStr=fixdt(1, 13, 0)  SampleTime=3.2e-05
  Iteration : Subsystem
  Iteration1 : Subsystem
  Iteration10 : Subsystem
  Iteration2 : Subsystem
  Iteration3 : Subsystem
  Iteration4 : Subsystem
  Iteration5 : Subsystem
  Iteration6 : Subsystem
  Iteration7 : Subsystem
  Iteration8 : Subsystem
  Iteration9 : Subsystem
  QuadrantMapper : Subsystem
  Terminator : Terminator
  cplx2reim : ComplexToRealImag  SampleTime=3.2e-05
  delayMatch{,1..23} (24 alike) : Delay  DelayLength=double(1)  InitialCondition=0  SampleTime=3.2e-05
  dtc : DataTypeConversion  OutDataTypeStr=fixdt(1, 13, 0)  SampleTime=3.2e-05
  dtc1 : DataTypeConversion  OutDataTypeStr=fixdt(1, 13, 0)  SampleTime=3.2e-05
  invert_reset : simulink/Logic and Bit Operations/Bitwise Operator  logicop=NOT  UseBitMask=off  BitMask=double(0)  BitMaskRealWorld=Real World Value
  muxMag : Switch  Criteria=u2 ~= 0  Threshold=double(0)  OutDataTypeStr=fixdt(1, 13, 0)  SampleTime=3.2e-05
  shift0 : Constant  VectorParams1D=off  OutDataTypeStr=fixdt(0, 5, 0)  SampleTime=3.2e-05
  shift1 : Constant  Value=2  VectorParams1D=off  OutDataTypeStr=fixdt(0, 5, 0)  SampleTime=3.2e-05
  shift10 : Constant  Value=11  VectorParams1D=off  OutDataTypeStr=fixdt(0, 5, 0)  SampleTime=3.2e-05
  shift2 : Constant  Value=3  VectorParams1D=off  OutDataTypeStr=fixdt(0, 5, 0)  SampleTime=3.2e-05
  shift3 : Constant  Value=4  VectorParams1D=off  OutDataTypeStr=fixdt(0, 5, 0)  SampleTime=3.2e-05
  shift4 : Constant  Value=5  VectorParams1D=off  OutDataTypeStr=fixdt(0, 5, 0)  SampleTime=3.2e-05
  shift5 : Constant  Value=6  VectorParams1D=off  OutDataTypeStr=fixdt(0, 5, 0)  SampleTime=3.2e-05
  shift6 : Constant  Value=7  VectorParams1D=off  OutDataTypeStr=fixdt(0, 5, 0)  SampleTime=3.2e-05
  shift7 : Constant  Value=8  VectorParams1D=off  OutDataTypeStr=fixdt(0, 5, 0)  SampleTime=3.2e-05
  shift8 : Constant  Value=9  VectorParams1D=off  OutDataTypeStr=fixdt(0, 5, 0)  SampleTime=3.2e-05
  shift9 : Constant  Value=10  VectorParams1D=off  OutDataTypeStr=fixdt(0, 5, 0)  SampleTime=3.2e-05
  Out1 : Outport
  Out2 : Outport  Port=2  VectorParamsAs1DForOutWhenUnconnected=off
  wires:
  muxMag/1 -> delayMatch23/1
  invert_reset/1 -> muxMag/2
  CSD Gain Factor/1 -> muxMag/3
  Initial_Val/1 -> muxMag/1
  Iteration10/1(xout) -> delayMatch22/1
  shift10/1 -> Iteration10/3(idx)
  Iteration10/2(yout) -> Terminator/1
  Iteration9/2(yout) -> delayMatch21/1
  Iteration9/1(xout) -> delayMatch20/1
  shift9/1 -> Iteration9/3(idx)
  Iteration8/2(yout) -> delayMatch19/1
  Iteration8/1(xout) -> delayMatch18/1
  shift8/1 -> Iteration8/3(idx)
  Iteration7/2(yout) -> delayMatch17/1
  Iteration7/1(xout) -> delayMatch16/1
  shift7/1 -> Iteration7/3(idx)
  Iteration6/2(yout) -> delayMatch15/1
  Iteration6/1(xout) -> delayMatch14/1
  shift6/1 -> Iteration6/3(idx)
  Iteration5/2(yout) -> delayMatch13/1
  Iteration5/1(xout) -> delayMatch12/1
  shift5/1 -> Iteration5/3(idx)
  Iteration4/2(yout) -> delayMatch11/1
  Iteration4/1(xout) -> delayMatch10/1
  shift4/1 -> Iteration4/3(idx)
  Iteration3/2(yout) -> delayMatch9/1
  Iteration3/1(xout) -> delayMatch8/1
  shift3/1 -> Iteration3/3(idx)
  Iteration2/2(yout) -> delayMatch7/1
  Iteration2/1(xout) -> delayMatch6/1
  shift2/1 -> Iteration2/3(idx)
  Iteration1/2(yout) -> delayMatch5/1
  Iteration1/1(xout) -> delayMatch4/1
  shift1/1 -> Iteration1/3(idx)
  Iteration/2(yout) -> delayMatch3/1
  Iteration/1(xout) -> delayMatch2/1
  shift0/1 -> Iteration/3(idx)
  dtc1/1 -> delayMatch1/1
  dtc/1 -> delayMatch/1
  cplx2reim/2 -> dtc1/1
  cplx2reim/1 -> dtc/1
  enable/1 -> Delay_ValidIn/1
  fft_data/1 -> cplx2reim/1
  delayMatch23/1 -> Out1/1
  Delay_ValidIn/1 -> invert_reset/1, DelayValidOut/1
  QuadrantMapper/2(yout) -> Iteration/2(yin)
  QuadrantMapper/1(xout) -> Iteration/1(xin)
  delayMatch1/1 -> QuadrantMapper/2(yin)
  delayMatch/1 -> QuadrantMapper/1(xin)
  delayMatch22/1 -> CSD Gain Factor/1
  delayMatch21/1 -> Iteration10/2(yin)
  delayMatch20/1 -> Iteration10/1(xin)
  delayMatch19/1 -> Iteration9/2(yin)
  delayMatch18/1 -> Iteration9/1(xin)
  delayMatch17/1 -> Iteration8/2(yin)
  delayMatch16/1 -> Iteration8/1(xin)
  delayMatch15/1 -> Iteration7/2(yin)
  delayMatch14/1 -> Iteration7/1(xin)
  delayMatch13/1 -> Iteration6/2(yin)
  delayMatch12/1 -> Iteration6/1(xin)
  delayMatch11/1 -> Iteration5/2(yin)
  delayMatch10/1 -> Iteration5/1(xin)
  delayMatch9/1 -> Iteration4/2(yin)
  delayMatch8/1 -> Iteration4/1(xin)
  delayMatch7/1 -> Iteration3/2(yin)
  delayMatch6/1 -> Iteration3/1(xin)
  delayMatch5/1 -> Iteration2/2(yin)
  delayMatch4/1 -> Iteration2/1(xin)
  delayMatch3/1 -> Iteration1/2(yin)
  delayMatch2/1 -> Iteration1/1(xin)
  DelayValidOut/1 -> Out2/1

== system gm_max_frequency_index/max_index_frequency/frequency_max/index_finder/for_each_instance21 ==
  fft_data : Inport  OutDataTypeStr=fixdt(1, 12, 0)  PortDimensions=1  SampleTime=3.2e-05
      settings: SignalType=complex
  enable : Inport  Port=2  OutDataTypeStr=boolean  PortDimensions=1  SampleTime=3.2e-05
  CSD Gain Factor : Gain  Gain="fi(0,0,13,13,\"hex\",\"1b7b\")"  ParamDataTypeStr=fixdt(0, 13, 13)  OutDataTypeStr=fixdt(1, 13, 0)  SampleTime=3.2e-05
  DelayValidOut : Delay  DelayLength=double(1)  InitialCondition=0  SampleTime=3.2e-05
  Delay_ValidIn : Delay  DelayLength=double(14)  InitialCondition=0  SampleTime=3.2e-05
  Initial_Val : Constant  Value=0  OutDataTypeStr=fixdt(1, 13, 0)  SampleTime=3.2e-05
  Iteration : Subsystem
  Iteration1 : Subsystem
  Iteration10 : Subsystem
  Iteration2 : Subsystem
  Iteration3 : Subsystem
  Iteration4 : Subsystem
  Iteration5 : Subsystem
  Iteration6 : Subsystem
  Iteration7 : Subsystem
  Iteration8 : Subsystem
  Iteration9 : Subsystem
  QuadrantMapper : Subsystem
  Terminator : Terminator
  cplx2reim : ComplexToRealImag  SampleTime=3.2e-05
  delayMatch{,1..23} (24 alike) : Delay  DelayLength=double(1)  InitialCondition=0  SampleTime=3.2e-05
  dtc : DataTypeConversion  OutDataTypeStr=fixdt(1, 13, 0)  SampleTime=3.2e-05
  dtc1 : DataTypeConversion  OutDataTypeStr=fixdt(1, 13, 0)  SampleTime=3.2e-05
  invert_reset : simulink/Logic and Bit Operations/Bitwise Operator  logicop=NOT  UseBitMask=off  BitMask=double(0)  BitMaskRealWorld=Real World Value
  muxMag : Switch  Criteria=u2 ~= 0  Threshold=double(0)  OutDataTypeStr=fixdt(1, 13, 0)  SampleTime=3.2e-05
  shift0 : Constant  VectorParams1D=off  OutDataTypeStr=fixdt(0, 5, 0)  SampleTime=3.2e-05
  shift1 : Constant  Value=2  VectorParams1D=off  OutDataTypeStr=fixdt(0, 5, 0)  SampleTime=3.2e-05
  shift10 : Constant  Value=11  VectorParams1D=off  OutDataTypeStr=fixdt(0, 5, 0)  SampleTime=3.2e-05
  shift2 : Constant  Value=3  VectorParams1D=off  OutDataTypeStr=fixdt(0, 5, 0)  SampleTime=3.2e-05
  shift3 : Constant  Value=4  VectorParams1D=off  OutDataTypeStr=fixdt(0, 5, 0)  SampleTime=3.2e-05
  shift4 : Constant  Value=5  VectorParams1D=off  OutDataTypeStr=fixdt(0, 5, 0)  SampleTime=3.2e-05
  shift5 : Constant  Value=6  VectorParams1D=off  OutDataTypeStr=fixdt(0, 5, 0)  SampleTime=3.2e-05
  shift6 : Constant  Value=7  VectorParams1D=off  OutDataTypeStr=fixdt(0, 5, 0)  SampleTime=3.2e-05
  shift7 : Constant  Value=8  VectorParams1D=off  OutDataTypeStr=fixdt(0, 5, 0)  SampleTime=3.2e-05
  shift8 : Constant  Value=9  VectorParams1D=off  OutDataTypeStr=fixdt(0, 5, 0)  SampleTime=3.2e-05
  shift9 : Constant  Value=10  VectorParams1D=off  OutDataTypeStr=fixdt(0, 5, 0)  SampleTime=3.2e-05
  Out1 : Outport
  Out2 : Outport  Port=2  VectorParamsAs1DForOutWhenUnconnected=off
  wires:
  muxMag/1 -> delayMatch23/1
  invert_reset/1 -> muxMag/2
  CSD Gain Factor/1 -> muxMag/3
  Initial_Val/1 -> muxMag/1
  Iteration10/1(xout) -> delayMatch22/1
  shift10/1 -> Iteration10/3(idx)
  Iteration10/2(yout) -> Terminator/1
  Iteration9/2(yout) -> delayMatch21/1
  Iteration9/1(xout) -> delayMatch20/1
  shift9/1 -> Iteration9/3(idx)
  Iteration8/2(yout) -> delayMatch19/1
  Iteration8/1(xout) -> delayMatch18/1
  shift8/1 -> Iteration8/3(idx)
  Iteration7/2(yout) -> delayMatch17/1
  Iteration7/1(xout) -> delayMatch16/1
  shift7/1 -> Iteration7/3(idx)
  Iteration6/2(yout) -> delayMatch15/1
  Iteration6/1(xout) -> delayMatch14/1
  shift6/1 -> Iteration6/3(idx)
  Iteration5/2(yout) -> delayMatch13/1
  Iteration5/1(xout) -> delayMatch12/1
  shift5/1 -> Iteration5/3(idx)
  Iteration4/2(yout) -> delayMatch11/1
  Iteration4/1(xout) -> delayMatch10/1
  shift4/1 -> Iteration4/3(idx)
  Iteration3/2(yout) -> delayMatch9/1
  Iteration3/1(xout) -> delayMatch8/1
  shift3/1 -> Iteration3/3(idx)
  Iteration2/2(yout) -> delayMatch7/1
  Iteration2/1(xout) -> delayMatch6/1
  shift2/1 -> Iteration2/3(idx)
  Iteration1/2(yout) -> delayMatch5/1
  Iteration1/1(xout) -> delayMatch4/1
  shift1/1 -> Iteration1/3(idx)
  Iteration/2(yout) -> delayMatch3/1
  Iteration/1(xout) -> delayMatch2/1
  shift0/1 -> Iteration/3(idx)
  dtc1/1 -> delayMatch1/1
  dtc/1 -> delayMatch/1
  cplx2reim/2 -> dtc1/1
  cplx2reim/1 -> dtc/1
  enable/1 -> Delay_ValidIn/1
  fft_data/1 -> cplx2reim/1
  delayMatch23/1 -> Out1/1
  Delay_ValidIn/1 -> invert_reset/1, DelayValidOut/1
  QuadrantMapper/2(yout) -> Iteration/2(yin)
  QuadrantMapper/1(xout) -> Iteration/1(xin)
  delayMatch1/1 -> QuadrantMapper/2(yin)
  delayMatch/1 -> QuadrantMapper/1(xin)
  delayMatch22/1 -> CSD Gain Factor/1
  delayMatch21/1 -> Iteration10/2(yin)
  delayMatch20/1 -> Iteration10/1(xin)
  delayMatch19/1 -> Iteration9/2(yin)
  delayMatch18/1 -> Iteration9/1(xin)
  delayMatch17/1 -> Iteration8/2(yin)
  delayMatch16/1 -> Iteration8/1(xin)
  delayMatch15/1 -> Iteration7/2(yin)
  delayMatch14/1 -> Iteration7/1(xin)
  delayMatch13/1 -> Iteration6/2(yin)
  delayMatch12/1 -> Iteration6/1(xin)
  delayMatch11/1 -> Iteration5/2(yin)
  delayMatch10/1 -> Iteration5/1(xin)
  delayMatch9/1 -> Iteration4/2(yin)
  delayMatch8/1 -> Iteration4/1(xin)
  delayMatch7/1 -> Iteration3/2(yin)
  delayMatch6/1 -> Iteration3/1(xin)
  delayMatch5/1 -> Iteration2/2(yin)
  delayMatch4/1 -> Iteration2/1(xin)
  delayMatch3/1 -> Iteration1/2(yin)
  delayMatch2/1 -> Iteration1/1(xin)
  DelayValidOut/1 -> Out2/1

== system gm_max_frequency_index/max_index_frequency/frequency_max/index_finder/for_each_instance22 ==
  fft_data : Inport  OutDataTypeStr=fixdt(1, 12, 0)  PortDimensions=1  SampleTime=3.2e-05
      settings: SignalType=complex
  enable : Inport  Port=2  OutDataTypeStr=boolean  PortDimensions=1  SampleTime=3.2e-05
  CSD Gain Factor : Gain  Gain="fi(0,0,13,13,\"hex\",\"1b7b\")"  ParamDataTypeStr=fixdt(0, 13, 13)  OutDataTypeStr=fixdt(1, 13, 0)  SampleTime=3.2e-05
  DelayValidOut : Delay  DelayLength=double(1)  InitialCondition=0  SampleTime=3.2e-05
  Delay_ValidIn : Delay  DelayLength=double(14)  InitialCondition=0  SampleTime=3.2e-05
  Initial_Val : Constant  Value=0  OutDataTypeStr=fixdt(1, 13, 0)  SampleTime=3.2e-05
  Iteration : Subsystem
  Iteration1 : Subsystem
  Iteration10 : Subsystem
  Iteration2 : Subsystem
  Iteration3 : Subsystem
  Iteration4 : Subsystem
  Iteration5 : Subsystem
  Iteration6 : Subsystem
  Iteration7 : Subsystem
  Iteration8 : Subsystem
  Iteration9 : Subsystem
  QuadrantMapper : Subsystem
  Terminator : Terminator
  cplx2reim : ComplexToRealImag  SampleTime=3.2e-05
  delayMatch{,1..23} (24 alike) : Delay  DelayLength=double(1)  InitialCondition=0  SampleTime=3.2e-05
  dtc : DataTypeConversion  OutDataTypeStr=fixdt(1, 13, 0)  SampleTime=3.2e-05
  dtc1 : DataTypeConversion  OutDataTypeStr=fixdt(1, 13, 0)  SampleTime=3.2e-05
  invert_reset : simulink/Logic and Bit Operations/Bitwise Operator  logicop=NOT  UseBitMask=off  BitMask=double(0)  BitMaskRealWorld=Real World Value
  muxMag : Switch  Criteria=u2 ~= 0  Threshold=double(0)  OutDataTypeStr=fixdt(1, 13, 0)  SampleTime=3.2e-05
  shift0 : Constant  VectorParams1D=off  OutDataTypeStr=fixdt(0, 5, 0)  SampleTime=3.2e-05
  shift1 : Constant  Value=2  VectorParams1D=off  OutDataTypeStr=fixdt(0, 5, 0)  SampleTime=3.2e-05
  shift10 : Constant  Value=11  VectorParams1D=off  OutDataTypeStr=fixdt(0, 5, 0)  SampleTime=3.2e-05
  shift2 : Constant  Value=3  VectorParams1D=off  OutDataTypeStr=fixdt(0, 5, 0)  SampleTime=3.2e-05
  shift3 : Constant  Value=4  VectorParams1D=off  OutDataTypeStr=fixdt(0, 5, 0)  SampleTime=3.2e-05
  shift4 : Constant  Value=5  VectorParams1D=off  OutDataTypeStr=fixdt(0, 5, 0)  SampleTime=3.2e-05
  shift5 : Constant  Value=6  VectorParams1D=off  OutDataTypeStr=fixdt(0, 5, 0)  SampleTime=3.2e-05
  shift6 : Constant  Value=7  VectorParams1D=off  OutDataTypeStr=fixdt(0, 5, 0)  SampleTime=3.2e-05
  shift7 : Constant  Value=8  VectorParams1D=off  OutDataTypeStr=fixdt(0, 5, 0)  SampleTime=3.2e-05
  shift8 : Constant  Value=9  VectorParams1D=off  OutDataTypeStr=fixdt(0, 5, 0)  SampleTime=3.2e-05
  shift9 : Constant  Value=10  VectorParams1D=off  OutDataTypeStr=fixdt(0, 5, 0)  SampleTime=3.2e-05
  Out1 : Outport
  Out2 : Outport  Port=2  VectorParamsAs1DForOutWhenUnconnected=off
  wires:
  muxMag/1 -> delayMatch23/1
  invert_reset/1 -> muxMag/2
  CSD Gain Factor/1 -> muxMag/3
  Initial_Val/1 -> muxMag/1
  Iteration10/1(xout) -> delayMatch22/1
  shift10/1 -> Iteration10/3(idx)
  Iteration10/2(yout) -> Terminator/1
  Iteration9/2(yout) -> delayMatch21/1
  Iteration9/1(xout) -> delayMatch20/1
  shift9/1 -> Iteration9/3(idx)
  Iteration8/2(yout) -> delayMatch19/1
  Iteration8/1(xout) -> delayMatch18/1
  shift8/1 -> Iteration8/3(idx)
  Iteration7/2(yout) -> delayMatch17/1
  Iteration7/1(xout) -> delayMatch16/1
  shift7/1 -> Iteration7/3(idx)
  Iteration6/2(yout) -> delayMatch15/1
  Iteration6/1(xout) -> delayMatch14/1
  shift6/1 -> Iteration6/3(idx)
  Iteration5/2(yout) -> delayMatch13/1
  Iteration5/1(xout) -> delayMatch12/1
  shift5/1 -> Iteration5/3(idx)
  Iteration4/2(yout) -> delayMatch11/1
  Iteration4/1(xout) -> delayMatch10/1
  shift4/1 -> Iteration4/3(idx)
  Iteration3/2(yout) -> delayMatch9/1
  Iteration3/1(xout) -> delayMatch8/1
  shift3/1 -> Iteration3/3(idx)
  Iteration2/2(yout) -> delayMatch7/1
  Iteration2/1(xout) -> delayMatch6/1
  shift2/1 -> Iteration2/3(idx)
  Iteration1/2(yout) -> delayMatch5/1
  Iteration1/1(xout) -> delayMatch4/1
  shift1/1 -> Iteration1/3(idx)
  Iteration/2(yout) -> delayMatch3/1
  Iteration/1(xout) -> delayMatch2/1
  shift0/1 -> Iteration/3(idx)
  dtc1/1 -> delayMatch1/1
  dtc/1 -> delayMatch/1
  cplx2reim/2 -> dtc1/1
  cplx2reim/1 -> dtc/1
  enable/1 -> Delay_ValidIn/1
  fft_data/1 -> cplx2reim/1
  delayMatch23/1 -> Out1/1
  Delay_ValidIn/1 -> invert_reset/1, DelayValidOut/1
  QuadrantMapper/2(yout) -> Iteration/2(yin)
  QuadrantMapper/1(xout) -> Iteration/1(xin)
  delayMatch1/1 -> QuadrantMapper/2(yin)
  delayMatch/1 -> QuadrantMapper/1(xin)
  delayMatch22/1 -> CSD Gain Factor/1
  delayMatch21/1 -> Iteration10/2(yin)
  delayMatch20/1 -> Iteration10/1(xin)
  delayMatch19/1 -> Iteration9/2(yin)
  delayMatch18/1 -> Iteration9/1(xin)
  delayMatch17/1 -> Iteration8/2(yin)
  delayMatch16/1 -> Iteration8/1(xin)
  delayMatch15/1 -> Iteration7/2(yin)
  delayMatch14/1 -> Iteration7/1(xin)
  delayMatch13/1 -> Iteration6/2(yin)
  delayMatch12/1 -> Iteration6/1(xin)
  delayMatch11/1 -> Iteration5/2(yin)
  delayMatch10/1 -> Iteration5/1(xin)
  delayMatch9/1 -> Iteration4/2(yin)
  delayMatch8/1 -> Iteration4/1(xin)
  delayMatch7/1 -> Iteration3/2(yin)
  delayMatch6/1 -> Iteration3/1(xin)
  delayMatch5/1 -> Iteration2/2(yin)
  delayMatch4/1 -> Iteration2/1(xin)
  delayMatch3/1 -> Iteration1/2(yin)
  delayMatch2/1 -> Iteration1/1(xin)
  DelayValidOut/1 -> Out2/1
